simulink model "simulink_group20"  (R2023a)
settings: Solver=FixedStepAuto  StartTime=0.0  StopTime=10.0  FixedStep=1e-3  RelTol=1e-3  EnableMultiTasking=on
undefined symbols (not defined in the file): D0, D1, D10, D11, D12, D13, D2, D3, D4, D5, D6, D7, D8, D9, PTA0, PTA1, PTA2, PTB23, PTB9, PTC16, PTC17, PTC2, PTC3, PTC4, PTD0, PTD1, PTD2, PTD3
libraries: frdmk64flib x19
settings Model: ExtModeTrigDuration=5  Creator=Karm  LastModifiedBy=Karm
settings OptimizationCC: EnhancedBackFolding=on  PassReuseOutputArgsAs=Individual arguments  ZeroExternalMemoryAtStartup=off  ZeroInternalMemoryAtStartup=off  MaxStackSize=64  OptimizeBlockOrder=speed  DifferentSizesBufferReuse=on  OptimizationCustomize=off  EfficientTunableParamExpr=on
settings DebuggingCC: ParameterTunabilityLossMsg=error
settings HardwareCC: ProdBitPerPointer=32  ProdBitPerSizeT=32  ProdBitPerPtrDiffT=32  ProdLargestAtomicInteger=Long  ProdLargestAtomicFloat=Double  ProdWordSize=32  ProdHWDeviceType=ARM Compatible->ARM Cortex
settings SFSimCC: MATLABDynamicMemAlloc=off
settings RTWCC: Description=Embedded Coder  SystemTargetFile=ert.tlc  HardwareBoard=NXP FRDM-K64F  TLCOptions="-aInlineSetEventsForThisBaseRateFcn=TLC_FALSE -aSuppressMultiTaskScheduler=TLC_FALSE  -aRateBasedStepFcn=0"  TemplateMakefile=ert_default_tmf  Toolchain=GNU Tools for ARM Embedded Processors
settings CodeAppCC: ForceParamTrailComments=on  IgnoreCustomStorageClasses=off  OperatorAnnotations=on  SimulinkDataObjDesc=on  SFDataObjDesc=on  InsertBlockDesc=on
settings ERTTargetCC: ExtModeTransport=4  ExtModeMexFile=sendToCommService

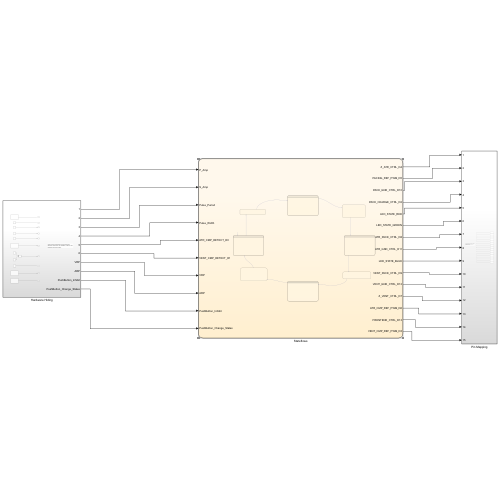
[thumbnail: Simulink's stored preview of the top-level diagram]
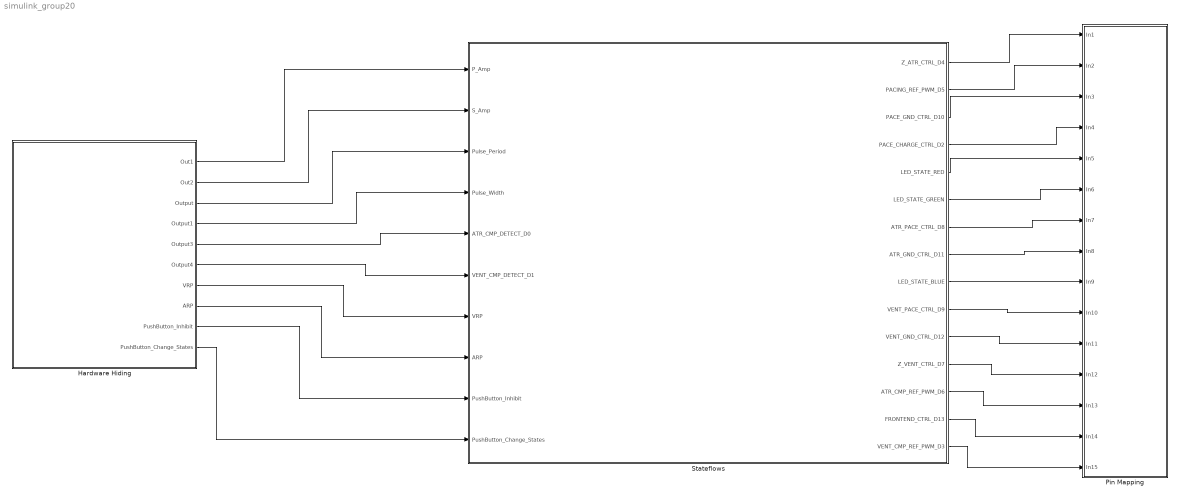
== system simulink_group20 ==
  Hardware Hiding : Subsystem
  Pin Mapping : Subsystem
  Stateflows : Stateflow chart  TreatAsAtomicUnit=on
      settings: PortSchema="{\"entries\":[{\"content\":{\"sides\":[{\"content\":{\"connectorIds\":[\"In1\",\"In9\",\"In2\",\"In8\",\"In3\",\"In4\",\"In5\",\"In6\",\"In7\",\"In10\"]},\"type\":\"ConnectorPlacement.EquallySpacedRectSide\",\"uuid\":\"fd7a65b5-6a9e-486c-b395-8752d247d110\"},{\"content\":{\"connectorIds\":[\"Out1\",\"Out2\",\"Out3\",\"Out4\",\"Out5\",\"Out6\",\"Out7\",\"Out8\",\"Out9\",\"Out10\",\"Out11\",\"Out12\",\"Out13\",\"Out14\",\"Out15\"],\"side\":\"RIGHT\"},\"type\":\"ConnectorPlacement.EquallySpacedRectSide\",\"uuid\":\"2771a934-b7e6-4717-9d0f-b17bdbdca872\"},{\"content\":{\"side\":\"TOP\"},\"type\":\"ConnectorPlacement.EquallySpacedRectSide\",\"uuid\":\"3a68066b-1574-4876-94b5-372b67bc25b8\"}]},\"type\":\"ConnectorPlacement.EquallySpacedConnector\",\"uuid\":\"cd95133d-7553-4814-ba78-1fbdc0c00507\"}],\"packageUris\":[\"http://schema.mathworks.com/mf0/Connector/R2020b\"],\"version\":\"1.0\"}"
  wires:
  Hardware Hiding/1(Out1) -> Stateflows/1(P_Amp)
  Hardware Hiding/2(Out2) -> Stateflows/9(S_Amp)
  Hardware Hiding/3(Output) -> Stateflows/2(Pulse_Period)
  Hardware Hiding/4(Output1) -> Stateflows/8(Pulse_Width)
  Hardware Hiding/5(Output3) -> Stateflows/3(ATR_CMP_DETECT_D0)
  Hardware Hiding/6(Output4) -> Stateflows/4(VENT_CMP_DETECT_D1)
  Hardware Hiding/7(VRP) -> Stateflows/5(VRP)
  Hardware Hiding/8(ARP) -> Stateflows/6(ARP)
  Hardware Hiding/9(PushButton_Inhibit) -> Stateflows/7(PushButton_Inhibit)
  Stateflows/1(Z_ATR_CTRL_D4) -> Pin Mapping/1(In1)
  Stateflows/2(PACING_REF_PWM_D5) -> Pin Mapping/2(In2)
  Stateflows/3(PACE_GND_CTRL_D10) -> Pin Mapping/3(In3)
  Stateflows/4(PACE_CHARGE_CTRL_D2) -> Pin Mapping/4(In4)
  Stateflows/5(LED_STATE_RED) -> Pin Mapping/5(In5)
  Stateflows/6(LED_STATE_GREEN) -> Pin Mapping/6(In6)
  Stateflows/7(ATR_PACE_CTRL_D8) -> Pin Mapping/7(In7)
  Stateflows/8(ATR_GND_CTRL_D11) -> Pin Mapping/8(In8)
  Stateflows/9(LED_STATE_BLUE) -> Pin Mapping/9(In9)
  Stateflows/10(VENT_PACE_CTRL_D9) -> Pin Mapping/10(In10)
  Stateflows/11(VENT_GND_CTRL_D12) -> Pin Mapping/11(In11)
  Stateflows/12(Z_VENT_CTRL_D7) -> Pin Mapping/12(In12)
  Stateflows/13(ATR_CMP_REF_PWM_D6) -> Pin Mapping/13(In13)
  Stateflows/14(FRONTEND_CTRL_D13) -> Pin Mapping/14(In14)
  Stateflows/15(VENT_CMP_REF_PWM_D3) -> Pin Mapping/15(In15)
  Hardware Hiding/10(PushButton_Change_States) -> Stateflows/10(PushButton_Change_States)

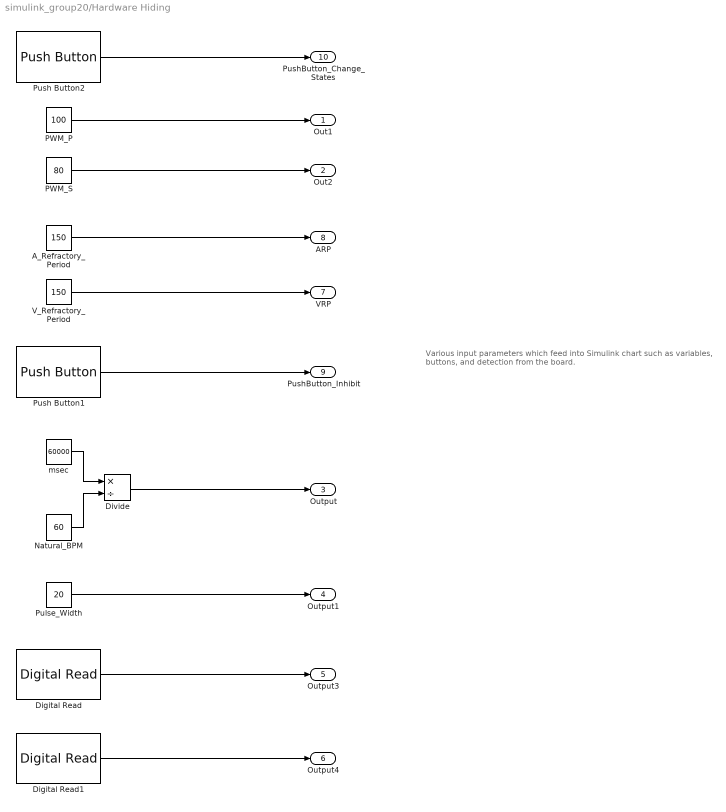
== system simulink_group20/Hardware Hiding ==
  note: Various input parameters which feed into
      | Simulink chart such as variables, buttons, and
      | detection from the board.
  A_Refractory_Period : Constant  Value=150
  Digital Read : frdmk64flib/Digital Read  Whichpin=PTC16 (D0)  SampleTime=-1
  Digital Read1 : frdmk64flib/Digital Read  Whichpin=PTC17 (D1)  SampleTime=-1
  Divide : Product  Inputs=*/
  Natural_BPM : Constant  Value=60
  PWM_P : Constant  Value=100
  PWM_S : Constant  Value=80
  Pulse_Width : Constant  Value=20  OutMin=[0]  OutMax=20  OutDataTypeStr=uint16  LockScale=on
  Push Button1 : frdmk64flib/Push Button  Whichswitch=SW3  SampleTime1=-1
  Push Button2 : frdmk64flib/Push Button  Whichswitch=SW2  SampleTime1=-1
  V_Refractory_Period : Constant  Value=150
  msec : Constant  Value=60000
  Out1 : Outport
  Out2 : Outport  Port=2
  Output : Outport  Port=3
  Output1 : Outport  Port=4
  Output3 : Outport  Port=5
  Output4 : Outport  Port=6
  VRP : Outport  Port=7
  ARP : Outport  Port=8
  PushButton_Inhibit : Outport  Port=9
  PushButton_Change_States : Outport  Port=10
  wires:
  PWM_S/1 -> Out2/1
  PWM_P/1 -> Out1/1
  Push Button1/1 -> PushButton_Inhibit/1
  V_Refractory_Period/1 -> VRP/1
  A_Refractory_Period/1 -> ARP/1
  Divide/1 -> Output/1
  msec/1 -> Divide/1
  Natural_BPM/1 -> Divide/2
  Pulse_Width/1 -> Output1/1
  Digital Read/1 -> Output3/1
  Digital Read1/1 -> Output4/1
  Push Button2/1 -> PushButton_Change_States/1

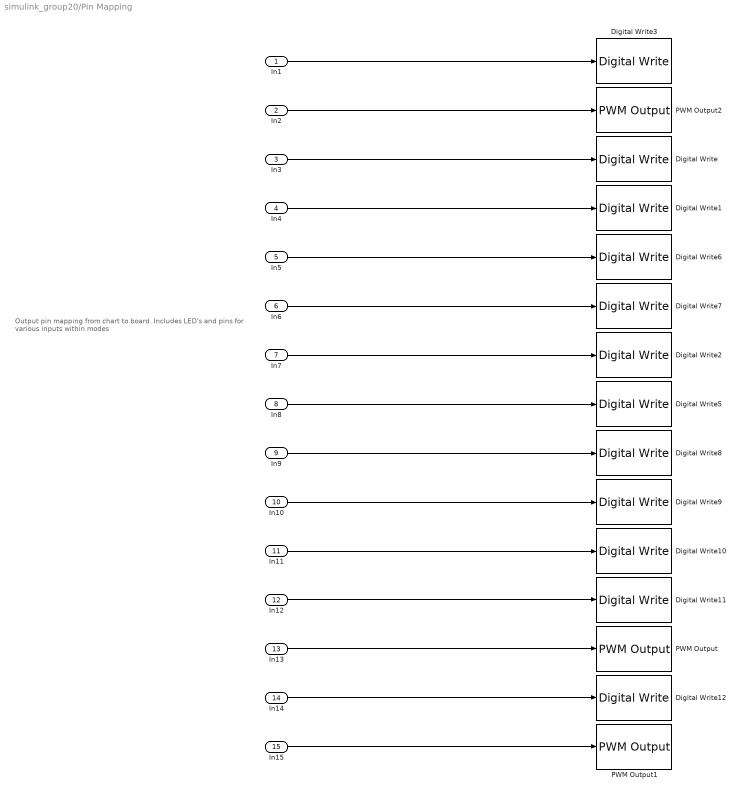
== system simulink_group20/Pin Mapping ==
  note: Output pin mapping from chart to board.
      | Includes LED's and pins for various
      | inputs within modes
  In1 : Inport
  In2 : Inport  Port=2
  In3 : Inport  Port=3
  In4 : Inport  Port=4
  In5 : Inport  Port=5
  In6 : Inport  Port=6
  In7 : Inport  Port=7
  In8 : Inport  Port=8
  In9 : Inport  Port=9
  In10 : Inport  Port=10
  In11 : Inport  Port=11
  In12 : Inport  Port=12
  In13 : Inport  Port=13
  In14 : Inport  Port=14
  In15 : Inport  Port=15
  Digital Write : frdmk64flib/Digital Write  Whichpin=PTD0 (D10)
  Digital Write1 : frdmk64flib/Digital Write  Whichpin=PTB9 (D2)
  Digital Write10 : frdmk64flib/Digital Write  Whichpin=PTD3 (D12)
  Digital Write11 : frdmk64flib/Digital Write  Whichpin=PTC3 (D7)
  Digital Write12 : frdmk64flib/Digital Write  Whichpin=PTD1 (D13)
  Digital Write2 : frdmk64flib/Digital Write  Whichpin=PTA0 (D8)
  Digital Write3 : frdmk64flib/Digital Write  Whichpin=PTB23 (D4)
  Digital Write5 : frdmk64flib/Digital Write  Whichpin=PTD2 (D11)
  Digital Write6 : frdmk64flib/Digital Write  Whichpin=RED_LED
  Digital Write7 : frdmk64flib/Digital Write  Whichpin=GREEN_LED
  Digital Write8 : frdmk64flib/Digital Write  Whichpin=BLUE_LED
  Digital Write9 : frdmk64flib/Digital Write  Whichpin=PTC4 (D9)
  PWM Output : frdmk64flib/PWM Output  Whichpin=PTC2 (D6)  InitialFrequency=2000  InitialDutyCycle=0
  PWM Output1 : frdmk64flib/PWM Output  Whichpin=PTA1 (D3)  InitialFrequency=2000  InitialDutyCycle=0
  PWM Output2 : frdmk64flib/PWM Output  Whichpin=PTA2 (D5)  InitialFrequency=2000  InitialDutyCycle=0
  wires:
  In6/1 -> Digital Write7/1
  In5/1 -> Digital Write6/1
  In1/1 -> Digital Write3/1
  In2/1 -> PWM Output2/1
  In4/1 -> Digital Write1/1
  In8/1 -> Digital Write5/1
  In7/1 -> Digital Write2/1
  In3/1 -> Digital Write/1
  In12/1 -> Digital Write11/1
  In9/1 -> Digital Write8/1
  In10/1 -> Digital Write9/1
  In11/1 -> Digital Write10/1
  In13/1 -> PWM Output/1
  In14/1 -> Digital Write12/1
  In15/1 -> PWM Output1/1

== stateflow chart simulink_group20/Stateflows ==
  state VVI
    note: Ventricular pacing, ventricular sensing, sensed intrinsic signal inhibits ventricular pacing
    state Pacing2
      % parameters laid out by documentation for Pacing
      entry:
      PACING_REF_PWM_D5 = P_Amp;
      PACE_CHARGE_CTRL_D2 = 0;
      VENT_PACE_CTRL_D9 = 1;
      VENT_GND_CTRL_D12 = 0;
      PACE_GND_CTRL_D10 = 1;
      Z_VENT_CTRL_D7 = 0;
      % LED visualization
      LED_STATE_RED = true;
      LED_STATE_BLUE = false;
      LED_STATE_GREEN=false;
    state Charging2
      % parameters laid out by documentation for Charging
      entry:
      PACING_REF_PWM_D5 = P_Amp;
      PACE_CHARGE_CTRL_D2 = 1;
      VENT_PACE_CTRL_D9 = 0;
      VENT_GND_CTRL_D12 = 1;
      PACE_GND_CTRL_D10 = 0;
      Z_VENT_CTRL_D7 = 0;
      FRONTEND_CTRL_D13 = 1;
      VENT_CMP_REF_PWM_D3 = S_Amp;
      % LED visualization
      LED_STATE_RED = false;
      LED_STATE_BLUE = true;
      LED_STATE_GREEN=false;
    (default) -> Charging2
    Pacing2 -> Charging2 : [after(Pulse_Width,msec)]
    Charging2 -> (junction 98) : after(VRP-Pulse_Width,msec)
    (junction 98) -> Pacing2 [order 2] : after(Pulse_Period-VRP,msec)[VENT_CMP_DETECT_D1 == 0 & PushButton_Inhibit == false]
    (junction 98) -> Charging2 [order 1] : [VENT_CMP_DETECT_D1 == 1 | PushButton_Inhibit == true]
  state Reset_VII_to_AOO
    entry:
    PACE_CHARGE_CTRL_D2 = 0;
    VENT_PACE_CTRL_D9 = 1;
    VENT_GND_CTRL_D12 = 0;
    PACE_GND_CTRL_D10 = 1;
    Z_VENT_CTRL_D7 = 0;
    % for demo purposes, nullifies actions from
    % previous state to move on to next state
  state Reset_VOO_to_VVI
    % for demo purposes, nullifies actions from
    % previous state to move on to next state
  state AOO
    note: Atrial pacing, no sensing
    state Charging1
      % parameters laid out by documentation for Charging
      entry:
      PACING_REF_PWM_D5 = P_Amp;
      PACE_CHARGE_CTRL_D2 = 1;
      PACE_GND_CTRL_D10 = 0;
      ATR_PACE_CTRL_D8 = 0;
      ATR_GND_CTRL_D11 = 1;
      Z_ATR_CTRL_D4 = 0;
      %LED visualization
      LED_STATE_RED = true;
      LED_STATE_GREEN = false;
      LED_STATE_BLUE = false;
    state Pacing1
      % parameters laid out by documentation for Pacing
      entry:
      PACING_REF_PWM_D5 = P_Amp;
      PACE_CHARGE_CTRL_D2 = 0;
      PACE_GND_CTRL_D10 = 1;
      ATR_PACE_CTRL_D8 = 1;
      ATR_GND_CTRL_D11 = 0;
      Z_ATR_CTRL_D4 = 0;
      %LED visualization
      LED_STATE_RED = false;
      LED_STATE_GREEN = true;
      LED_STATE_BLUE = false;
    (default) -> Charging1
    Charging1 -> Pacing1 : [after(Pulse_Period-Pulse_Width,msec)]
    Pacing1 -> Charging1 : [after(Pulse_Width,msec)]
  state VOO
    state Charging
      % parameters laid out by documentation for Charging
      entry:
      PACING_REF_PWM_D5 = P_Amp;
      PACE_CHARGE_CTRL_D2 = 1;
      PACE_GND_CTRL_D10 = 0;
      Z_VENT_CTRL_D7 = 0;
      VENT_GND_CTRL_D12 = 1;
      VENT_PACE_CTRL_D9 = 0;
      % LED visualization
      LED_STATE_RED = false;
      LED_STATE_BLUE = true;
      LED_STATE_GREEN=false;
    state Pacing
      % parameters laid out by documentation for Pacing
      entry:
      PACING_REF_PWM_D5 = P_Amp;
      PACE_CHARGE_CTRL_D2 = 0;
      PACE_GND_CTRL_D10 = 1;
      Z_VENT_CTRL_D7 = 0;
      VENT_GND_CTRL_D12 = 0;
      VENT_PACE_CTRL_D9 = 1;
      %LED visualization
      LED_STATE_RED = true;
      LED_STATE_BLUE = false;
      LED_STATE_GREEN=false;
    note: Ventricular pacing, no sensing
    (default) -> Charging
    Charging -> Pacing : [after(Pulse_Period-Pulse_Width,msec)]
    Pacing -> Charging : [after(Pulse_Width,msec)]
  state Reset_AAI_to_VOO
    entry:
    PACE_CHARGE_CTRL_D2=0;
    ATR_PACE_CTRL_D8= 1;
    ATR_GND_CTRL_D11= 0;
    PACE_GND_CTRL_D10=1;
    Z_ATR_CTRL_D4=0;
    % for demo purposes, nullifies actions from
    % previous state to move on to next state
  state Reset_AOO_to_AAI
    % for demo purposes, nullifies actions from
    % previous state to move on to next state
  state AAI
    state Charging3
      % parameters laid out by documentation for Charging
      entry:
      PACING_REF_PWM_D5 = P_Amp;
      PACE_CHARGE_CTRL_D2=1;
      ATR_PACE_CTRL_D8= 0;
      ATR_GND_CTRL_D11= 1;
      PACE_GND_CTRL_D10=0;
      Z_ATR_CTRL_D4=0;
      FRONTEND_CTRL_D13 = 1;
      ATR_CMP_REF_PWM_D6 = S_Amp;
      % LED visualization
      LED_STATE_RED=true;
      LED_STATE_GREEN=false;
      LED_STATE_BLUE = false;
    state Pacing3
      % parameters laid out by documentation for Pacing
      entry:
      PACING_REF_PWM_D5 = P_Amp;
      PACE_CHARGE_CTRL_D2=0;
      ATR_PACE_CTRL_D8= 1;
      ATR_GND_CTRL_D11= 0;
      PACE_GND_CTRL_D10=1;
      Z_ATR_CTRL_D4=0;
      % LED visualization
      LED_STATE_RED=false;
      LED_STATE_GREEN=true;
      LED_STATE_BLUE = false;
    note: Atrial pacing, atrial sensing, sensed intrinsic signal inhibits atrial pacing
    (default) -> Charging3
    (junction 72) -> Charging3 [order 1] : [ATR_CMP_DETECT_D0 == 1 | PushButton_Inhibit == true]
    Charging3 -> (junction 72) : after(ARP-Pulse_Width, msec)
    (junction 72) -> Pacing3 [order 2] : after(Pulse_Period-ARP,msec)[ATR_CMP_DETECT_D0 == 0 & PushButton_Inhibit == false]
    Pacing3 -> Charging3 : after(Pulse_Width,msec)
  VVI -> Reset_VII_to_AOO : after(Pulse_Period,msec)[PushButton_Change_States == true]
  Reset_VOO_to_VVI -> VVI : after(Pulse_Period,msec)[PushButton_Change_States == true]
  VOO -> Reset_VOO_to_VVI : after(Pulse_Period,msec)[PushButton_Change_States == true]
  Reset_VII_to_AOO -> AOO : after(Pulse_Period,msec)[PushButton_Change_States == true]
  (default) -> VOO
  AOO -> Reset_AOO_to_AAI : after(Pulse_Period,msec)[PushButton_Change_States == true]
  Reset_AAI_to_VOO -> VOO : after(Pulse_Period,msec)[PushButton_Change_States == true]
  Reset_AOO_to_AAI -> AAI : after(Pulse_Period,msec)[PushButton_Change_States == true]
  AAI -> Reset_AAI_to_VOO : after(Pulse_Period,msec)[PushButton_Change_States == true]
  data: P_Amp input; Pulse_Period input; ATR_CMP_DETECT_D0 input; VENT_CMP_DETECT_D1 input; VRP input; ARP input; PushButton_Inhibit input; Pulse_Width input; S_Amp input; Z_ATR_CTRL_D4 output; PACING_REF_PWM_D5 output; PACE_GND_CTRL_D10 output; PACE_CHARGE_CTRL_D2 output; LED_STATE_RED output; LED_STATE_GREEN output; ATR_PACE_CTRL_D8 output; ATR_GND_CTRL_D11 output; LED_STATE_BLUE output; VENT_PACE_CTRL_D9 output; VENT_GND_CTRL_D12 output; Z_VENT_CTRL_D7 output; ATR_CMP_REF_PWM_D6 output; FRONTEND_CTRL_D13 output; VENT_CMP_REF_PWM_D3 output; PushButton_Change_States input; State local
